simulink model "InterModel_TX"  (Simulink 7.4)
settings: Solver=FixedStepDiscrete  SolverMode=SingleTasking  StartTime=0.0  StopTime=inf  FixedStep=.02  RelTol=1e-3
settings Model: Creator=fwornle  LastModifiedBy=fw  ExtModeTrigDuration=500
settings ConfigSet: Description=rtmc9s12target_R2008a
settings DataIOCC: SignalLoggingName=sigsOut
settings OptimizationCC: BooleanDataType=off  InitFltsAndDblsToZero=on
settings DebuggingCC: SaveWithParameterizedLinksMsg=none  SignalResolutionControl=TryResolveAllWithWarning  SolverPrmCheckMsg=none  MultiTaskDSMMsg=warning  MultiTaskCondExecSysMsg=none  StrictBusMsg=None
settings HardwareCC: ProdBitPerInt=16  ProdEndianess=BigEndian  ProdWordSize=16  ProdHWDeviceType=Motorola HC12  TargetHWDeviceType=32-bit Generic  ProdEqTarget=off
settings RTWCC: GenerateMakefile=off  TemplateMakefile=grt_msvc.tmf  Description="Visual C/C++ Project Makefile only for the \"grt\" target"  ProcessScript=grt_make_rtw_hook  IncludeERTFirstTime=on
settings GRTTargetCC: TargetFcnLib=ansi_tfl_tmw.mat

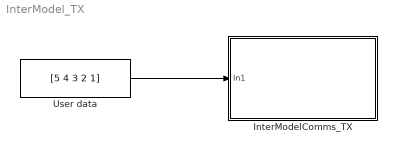
== system InterModel_TX ==
  InterModelComms_TX : Subsystem  Tag=mcTarget_freePortCommsRX  mask{sampletime=0.1, channel=0, buf_size=5, data_type=UINT8}
      mask prompts: sampletime "Sample time"; channel "Channel number"; buf_size "Number of elements"; data_type "Data Type"
      mask init:
      | [buf_sizestr, channelstr, data_type_str, sampletime_str] = mbc_intermodeltxd(sampletime, channel, buf_size, data_type);
      mask Help: web('freePortComms_rxd.html');
      mask StyleString: edit,edit,edit,popup(SINGLE|INT8|UINT8|INT16|UINT16|INT32|UINT32|BOOLEAN)
      mask Display: fprintf('Transmit %s element(s)\nChannel: %s\nData type: %s\n Sample rate: %s', buf_sizestr, channelstr, data_type_str, sampletime_str)
  User data : Constant  Value=[5 4 3 2 1]  OutDataType=sfix(16)  OutScaling=2^0
  wires:
  User data/1 -> InterModelComms_TX/1(In1)

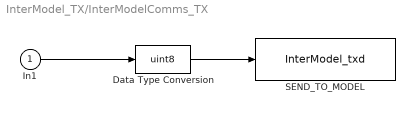
== system InterModel_TX/InterModelComms_TX ==
  In1 : Inport  OutDataType=sfix(16)  OutScaling=2^0
  Data Type Conversion : DataTypeConversion  OutDataTypeMode=uint8  OutDataType=sfix(16)  OutScaling=2^0  OutDataTypeStr=uint8  SaturateOnIntegerOverflow=on  RndMeth=Zero
  SEND_TO_MODEL : S-Function  Tag=mcTarget_freePortCommsRX  FunctionName=InterModel_txd  Parameters=sampletime, channel, buf_size, data_type  EnableBusSupport=off
  wires:
  In1/1 -> Data Type Conversion/1
  Data Type Conversion/1 -> SEND_TO_MODEL/1
